simulink model "Quadcopter_Modelling_WILSEL_SR"  (R2024b)
settings: Solver=VariableStepAuto  StartTime=0.0  StopTime=10.0  RelTol=1e-3
undefined symbols (not defined in the file): g, Ixx, Iyy, Izz, l, m
settings Model: Creator=ros  LastModifiedBy=ros

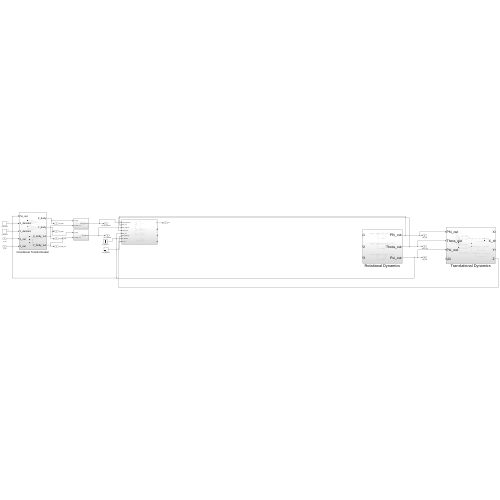
[thumbnail: Simulink's stored preview of the top-level diagram]
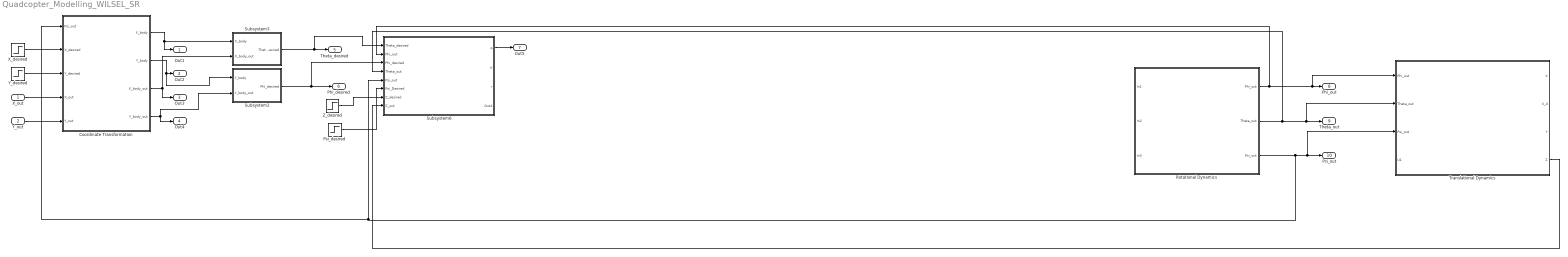
== system Quadcopter_Modelling_WILSEL_SR ==
  X_out : Inport
  Y_out : Inport  Port=2
  Coordinate Transformation : Subsystem
  Psi_desired : Step  After=0  SampleTime=0
  Rotational Dynamics : Subsystem
  Subsystem2 : Subsystem
  Subsystem3 : Subsystem
  Subsystem6 : Subsystem
  Translational Dynamics : Subsystem
  X_desired : Step  SampleTime=0
  Y_desired : Step  SampleTime=0
  Z_desired : Step  SampleTime=0
  Out1 : Outport  SignalName=X_body
  Out2 : Outport  Port=2  SignalName=Y_body
  Out3 : Outport  Port=3  SignalName=X_body_out
  Out4 : Outport  Port=4  SignalName=Y_body_out
  Theta_desired : Outport  Port=5
  Phi_desired : Outport  Port=6
  Out5 : Outport  Port=7  SignalName=U1
  Phi_out : Outport  Port=8
  Theta_out : Outport  Port=9
  Psi_out : Outport  Port=10
  wires:
  X_desired/1 -> Coordinate Transformation/2(X_desired)
  Y_desired/1 -> Coordinate Transformation/3(Y_desired)
  X_out/1 -> Coordinate Transformation/4(X_out)
  Y_out/1 -> Coordinate Transformation/5(Y_out)
  Coordinate Transformation/1(X_body) -> Out1/1, Subsystem3/1(X_body)
  Coordinate Transformation/2(Y_body) -> Subsystem2/1(Y_body), Out2/1
  Coordinate Transformation/4(Y_body_out) -> Out4/1, Subsystem2/2(Y_body_out)
  Coordinate Transformation/3(X_body_out) -> Out3/1, Subsystem3/2(X_body_out)
  Subsystem2/1(Phi_desired) -> Phi_desired/1, Subsystem6/3(Phi_desired)
  Subsystem3/1(Theta_desired) -> Subsystem6/1(Theta_desired), Theta_desired/1
  Rotational Dynamics/1(Phi_out) -> Subsystem6/2(Phi_out), Translational Dynamics/1(Phi_out), Phi_out/1
  Rotational Dynamics/2(Theta_out) -> Subsystem6/4(Theta_out), Translational Dynamics/2(Theta_out), Theta_out/1
  Rotational Dynamics/3(Psi_out) -> Coordinate Transformation/1(Psi_out), Subsystem6/5(Psi_out), Translational Dynamics/3(Psi_out), Psi_out/1
  Psi_desired/1 -> Subsystem6/6(Psi_Desired)
  Z_desired/1 -> Subsystem6/7(Z_desired)
  Subsystem6/1(q) -> Out5/1
  Translational Dynamics/4(Z) -> Subsystem6/8(Z_out)

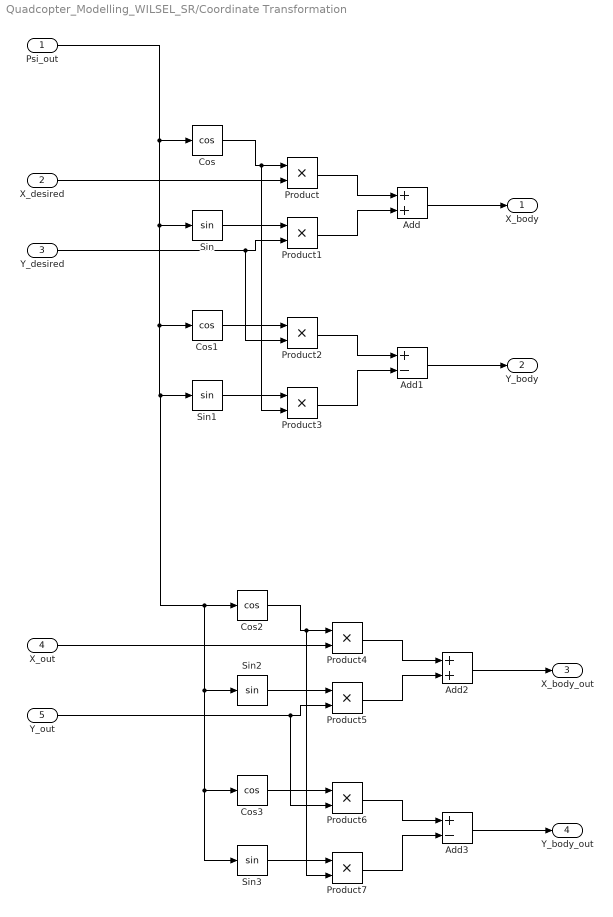
== system Quadcopter_Modelling_WILSEL_SR/Coordinate Transformation ==
  Psi_out : Inport
  X_desired : Inport  Port=2
  Y_desired : Inport  Port=3
  X_out : Inport  Port=4
  Y_out : Inport  Port=5
  Add : Sum
  Add1 : Sum  Inputs=+-
  Add2 : Sum
  Add3 : Sum  Inputs=+-
  Cos{,1..3} (4 alike) : Trigonometry  Operator=cos
  Product{,1..7} (8 alike) : Product
  Sin{,1..3} (4 alike) : Trigonometry
  X_body : Outport
  Y_body : Outport  Port=2
  X_body_out : Outport  Port=3
  Y_body_out : Outport  Port=4
  wires:
  Cos2/1 -> Product7/2, Product4/1
  Add3/1 -> Y_body_out/1
  Product7/1 -> Add3/2
  Sin2/1 -> Product5/1
  Add2/1 -> X_body_out/1
  Sin1/1 -> Product3/1
  Y_desired/1 -> Product2/2, Product1/2
  Cos3/1 -> Product6/1
  Product6/1 -> Add3/1
  X_desired/1 -> Product/2
  Product1/1 -> Add/2
  Product3/1 -> Add1/2
  Cos/1 -> Product3/2, Product/1
  Product5/1 -> Add2/2
  Sin/1 -> Product1/1
  Psi_out/1 -> Sin3/1, Cos3/1, Sin2/1, Cos2/1, Sin1/1, Cos1/1, Sin/1, Cos/1
  Sin3/1 -> Product7/1
  Add1/1 -> Y_body/1
  Product/1 -> Add/1
  Add/1 -> X_body/1
  X_out/1 -> Product4/2
  Product4/1 -> Add2/1
  Product2/1 -> Add1/1
  Y_out/1 -> Product6/2, Product5/2
  Cos1/1 -> Product2/1

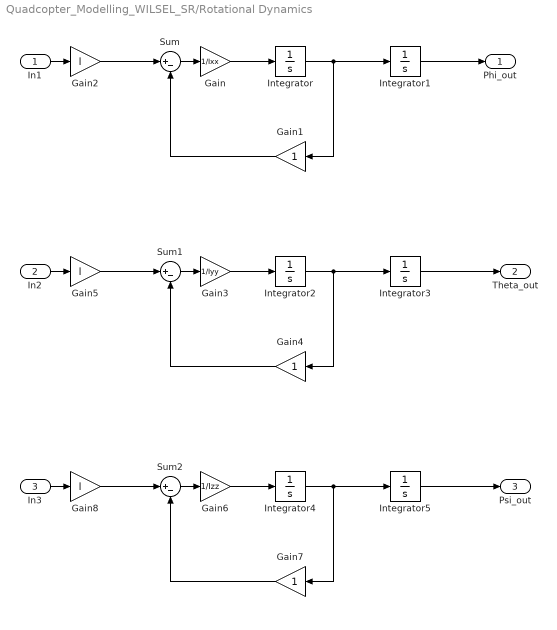
== system Quadcopter_Modelling_WILSEL_SR/Rotational Dynamics ==
  In1 : Inport
  In2 : Inport  Port=2
  In3 : Inport  Port=3
  Gain : Gain  Gain=1/Ixx
  Gain1 : Gain
  Gain2 : Gain  Gain=l
  Gain3 : Gain  Gain=1/Iyy
  Gain4 : Gain
  Gain5 : Gain  Gain=l
  Gain6 : Gain  Gain=1/Izz
  Gain7 : Gain
  Gain8 : Gain  Gain=l
  Integrator{,1..5} (6 alike) : Integrator
  Sum : Sum  Inputs=|+-
  Sum1 : Sum  Inputs=|+-
  Sum2 : Sum  Inputs=|+-
  Phi_out : Outport
  Theta_out : Outport  Port=2
  Psi_out : Outport  Port=3
  wires:
  Gain7/1 -> Sum2/2
  Gain5/1 -> Sum1/1
  Gain4/1 -> Sum1/2
  Gain3/1 -> Integrator2/1
  Gain1/1 -> Sum/2
  Sum/1 -> Gain/1
  In3/1 -> Gain8/1
  Integrator/1 -> Gain1/1, Integrator1/1
  Gain/1 -> Integrator/1
  In1/1 -> Gain2/1
  Integrator3/1 -> Theta_out/1
  Sum1/1 -> Gain3/1
  Integrator5/1 -> Psi_out/1
  Integrator1/1 -> Phi_out/1
  Gain8/1 -> Sum2/1
  Gain6/1 -> Integrator4/1
  Integrator4/1 -> Gain7/1, Integrator5/1
  In2/1 -> Gain5/1
  Sum2/1 -> Gain6/1
  Integrator2/1 -> Gain4/1, Integrator3/1
  Gain2/1 -> Sum/1

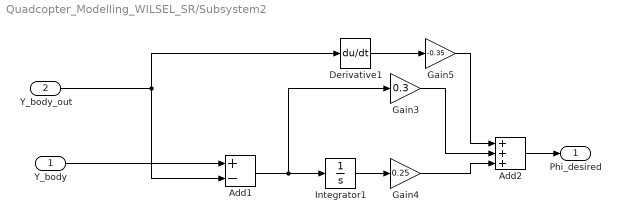
== system Quadcopter_Modelling_WILSEL_SR/Subsystem2 ==
  Y_body : Inport
  Y_body_out : Inport  Port=2
  Add1 : Sum  Inputs=+-
  Add2 : Sum  Inputs=+++
  Derivative1 : Derivative
  Gain3 : Gain  Gain=0.3
  Gain4 : Gain  Gain=0.25
  Gain5 : Gain  Gain=-0.35
  Integrator1 : Integrator
  Phi_desired : Outport
  wires:
  Add2/1 -> Phi_desired/1
  Derivative1/1 -> Gain5/1
  Gain5/1 -> Add2/1
  Gain3/1 -> Add2/2
  Add1/1 -> Gain3/1, Integrator1/1
  Integrator1/1 -> Gain4/1
  Gain4/1 -> Add2/3
  Y_body/1 -> Add1/1
  Y_body_out/1 -> Add1/2, Derivative1/1

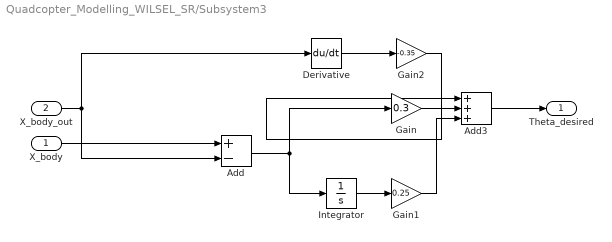
== system Quadcopter_Modelling_WILSEL_SR/Subsystem3 ==
  X_body : Inport
  X_body_out : Inport  Port=2
  Add : Sum  Inputs=+-
  Add3 : Sum  Inputs=+++
  Derivative : Derivative
  Gain : Gain  Gain=0.3
  Gain1 : Gain  Gain=0.25
  Gain2 : Gain  Gain=-0.35
  Integrator : Integrator
  Theta_desired : Outport
  wires:
  Gain2/1 -> Add3/1
  Derivative/1 -> Gain2/1
  Add3/1 -> Theta_desired/1
  Gain1/1 -> Add3/3
  X_body/1 -> Add/1
  Add/1 -> Gain/1, Integrator/1
  Integrator/1 -> Gain1/1
  X_body_out/1 -> Add/2, Derivative/1
  Gain/1 -> Add3/2

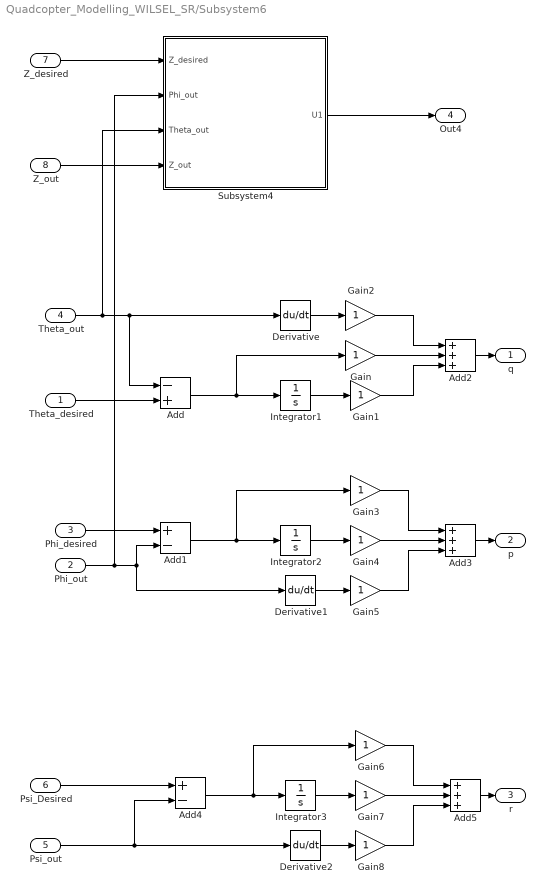
== system Quadcopter_Modelling_WILSEL_SR/Subsystem6 ==
  Theta_desired : Inport
  Phi_out : Inport  Port=2
  Phi_desired : Inport  Port=3
  Theta_out : Inport  Port=4
  Psi_out : Inport  Port=5
  Psi_Desired : Inport  Port=6
  Z_desired : Inport  Port=7
  Z_out : Inport  Port=8
  Add : Sum  Inputs=-+
  Add1 : Sum  Inputs=+-
  Add2 : Sum  Inputs=+++
  Add3 : Sum  Inputs=+++
  Add4 : Sum  Inputs=+-
  Add5 : Sum  Inputs=+++
  Derivative : Derivative
  Derivative1 : Derivative
  Derivative2 : Derivative
  Gain{,1..8} (9 alike) : Gain
  Integrator1 : Integrator
  Integrator2 : Integrator
  Integrator3 : Integrator
  Subsystem4 : Subsystem
  q : Outport
  p : Outport  Port=2
  r : Outport  Port=3
  Out4 : Outport  Port=4
  wires:
  Derivative/1 -> Gain2/1
  Integrator1/1 -> Gain1/1
  Gain2/1 -> Add2/1
  Derivative1/1 -> Gain5/1
  Gain3/1 -> Add3/1
  Gain8/1 -> Add5/3
  Gain5/1 -> Add3/3
  Add1/1 -> Gain3/1, Integrator2/1
  Add/1 -> Gain/1, Integrator1/1
  Integrator3/1 -> Gain7/1
  Theta_desired/1 -> Add/2
  Psi_out/1 -> Add4/2, Derivative2/1
  Psi_Desired/1 -> Add4/1
  Add2/1 -> q/1
  Phi_desired/1 -> Add1/1
  Gain1/1 -> Add2/3
  Add3/1 -> p/1
  Gain7/1 -> Add5/2
  Add4/1 -> Gain6/1, Integrator3/1
  Derivative2/1 -> Gain8/1
  Gain6/1 -> Add5/1
  Gain/1 -> Add2/2
  Add5/1 -> r/1
  Integrator2/1 -> Gain4/1
  Gain4/1 -> Add3/2
  Subsystem4/1(U1) -> Out4/1
  Z_desired/1 -> Subsystem4/1(Z_desired)
  Z_out/1 -> Subsystem4/4(Z_out)
  Phi_out/1 -> Subsystem4/2(Phi_out), Derivative1/1, Add1/2
  Theta_out/1 -> Subsystem4/3(Theta_out), Add/1, Derivative/1

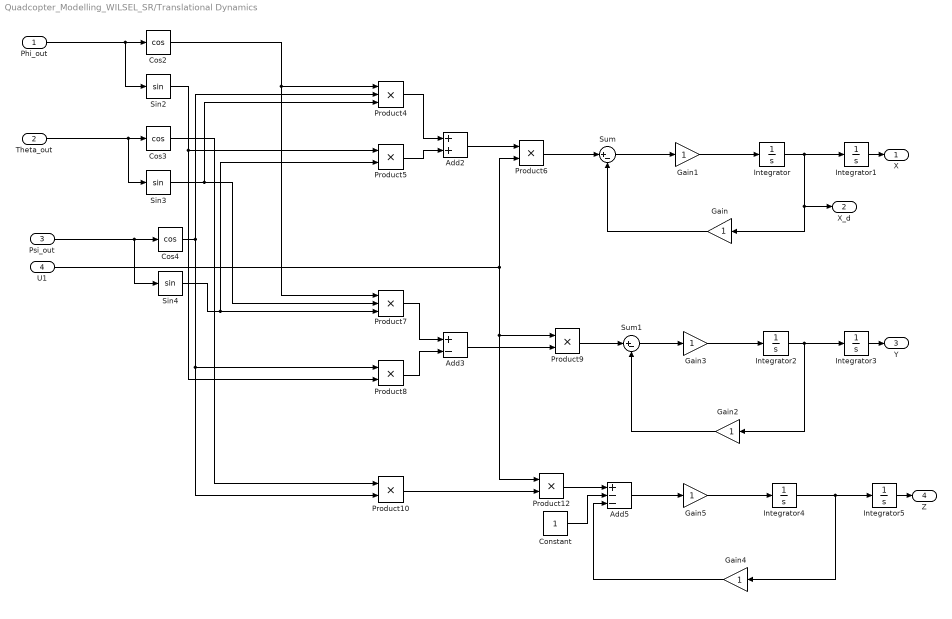
== system Quadcopter_Modelling_WILSEL_SR/Translational Dynamics ==
  Phi_out : Inport
  Theta_out : Inport  Port=2
  Psi_out : Inport  Port=3
  U1 : Inport  Port=4
  Add2 : Sum
  Add3 : Sum  Inputs=+-
  Add5 : Sum  Inputs=+--
  Constant : Constant
  Cos2 : Trigonometry  Operator=cos
  Cos3 : Trigonometry  Operator=cos
  Cos4 : Trigonometry  Operator=cos
  Gain{,1..5} (6 alike) : Gain
  Integrator{,1..5} (6 alike) : Integrator
  Product{5..6,8..10,12} (6 alike) : Product
  Product4 : Product  Inputs=3
  Product7 : Product  Inputs=3
  Sin2 : Trigonometry
  Sin3 : Trigonometry
  Sin4 : Trigonometry
  Sum : Sum  Inputs=|+-
  Sum1 : Sum  Inputs=|+-
  X : Outport
  X_d : Outport  Port=2
  Y : Outport  Port=3
  Z : Outport  Port=4
  wires:
  Product10/1 -> Product12/2
  Add2/1 -> Product6/1
  Product8/1 -> Add3/2
  Product6/1 -> Sum/1
  Gain3/1 -> Integrator2/1
  Gain1/1 -> Integrator/1
  Integrator1/1 -> X/1
  Product12/1 -> Add5/1
  Product7/1 -> Add3/1
  Theta_out/1 -> Sin3/1, Cos3/1
  Gain/1 -> Sum/2
  Integrator4/1 -> Gain4/1, Integrator5/1
  Cos3/1 -> Product10/1
  Constant/1 -> Add5/2
  Gain4/1 -> Add5/3
  Sin2/1 -> Product5/1, Product8/2
  Sum/1 -> Gain1/1
  Sin4/1 -> Product5/2, Product7/3
  Gain5/1 -> Integrator4/1
  Integrator3/1 -> Y/1
  Add5/1 -> Gain5/1
  Product5/1 -> Add2/2
  Integrator5/1 -> Z/1
  Cos4/1 -> Product4/2, Product10/2, Product8/1
  Integrator2/1 -> Gain2/1, Integrator3/1
  Sin3/1 -> Product4/3, Product7/2
  Sum1/1 -> Gain3/1
  Add3/1 -> Product9/2
  Phi_out/1 -> Sin2/1, Cos2/1
  Product9/1 -> Sum1/1
  U1/1 -> Product12/1, Product9/1, Product6/2
  Psi_out/1 -> Sin4/1, Cos4/1
  Product4/1 -> Add2/1
  Cos2/1 -> Product4/1, Product7/1
  Gain2/1 -> Sum1/2
  Integrator/1 -> X_d/1, Gain/1, Integrator1/1

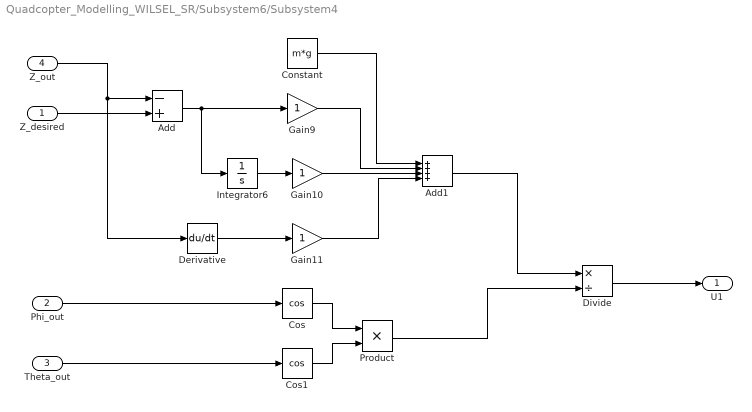
== system Quadcopter_Modelling_WILSEL_SR/Subsystem6/Subsystem4 ==
  Z_desired : Inport
  Phi_out : Inport  Port=2
  Theta_out : Inport  Port=3
  Z_out : Inport  Port=4
  Add : Sum  Inputs=-+
  Add1 : Sum  Inputs=++++
  Constant : Constant  Value=m*g
  Cos : Trigonometry  Operator=cos
  Cos1 : Trigonometry  Operator=cos
  Derivative : Derivative
  Divide : Product  Inputs=*/
  Gain10 : Gain
  Gain11 : Gain
  Gain9 : Gain
  Integrator6 : Integrator
  Product : Product
  U1 : Outport
  wires:
  Gain10/1 -> Add1/3
  Derivative/1 -> Gain11/1
  Add1/1 -> Divide/1
  Phi_out/1 -> Cos/1
  Gain9/1 -> Add1/2
  Theta_out/1 -> Cos1/1
  Constant/1 -> Add1/1
  Cos1/1 -> Product/2
  Add/1 -> Integrator6/1, Gain9/1
  Divide/1 -> U1/1
  Integrator6/1 -> Gain10/1
  Product/1 -> Divide/2
  Z_out/1 -> Derivative/1, Add/1
  Cos/1 -> Product/1
  Gain11/1 -> Add1/4
  Z_desired/1 -> Add/2
